simulink model "qa_old_models"  (Simulink 7.3)
settings: Solver=ode45  StartTime=0.0  StopTime=10.0  RelTol=1e-3
values from neighbouring files (symbols this model uses):
  fixpt_adder_out_bitwidth = w    (= 24)    [one_bit_control.m]
  fixpt_adder_out_position = d    (= 16)    [one_bit_control.m]
settings Model: Creator=kunal  LastModifiedBy=kunal

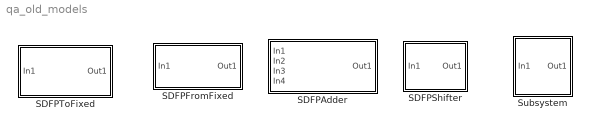
== system qa_old_models ==
  SDFPAdder : Subsystem  mask{in_bitwidth=32, in_fp_position=8, out_bitwidth=32, out_fp_position=8}
      mask prompts: in_bitwidth "Input Bitwidth"; in_fp_position "Input Point Position"; out_bitwidth "Output Bitwidth"; out_fp_position "Output Point Position"
      mask Display: disp(['+\nSDFP'])
  SDFPFromFixed : Subsystem  mask{bitwidth=32, fp_position=16}
      mask prompts: bitwidth "Input Bitwidth"; fp_position "Input Point Position"
      mask Display: disp('Fixed -> Float');
  SDFPShifter : Subsystem  mask{shift_amount=1}
      mask init:
      | if(shift_amount > 0)
      |     dispval=sprintf('<< %d',shift_amount);
      | else
      |     dispval=sprintf('>> %d',-shift_amount);
      | end
      mask Display: disp(dispval);
  SDFPToFixed : Subsystem  mask{bitwidth=fixpt_adder_out_bitwidth, fp_position=fixpt_adder_out_position}
      mask prompts: bitwidth "Output Bitwidth"; fp_position "Output Point Position"
      mask Display: disp('Float -> Fixed')
  Subsystem : Subsystem  mask{gain=1.52, bitwidth=32, fp_position=16}
      mask prompts: bitwidth "Output Bitwidth"; fp_position "Output Point Position"
      mask Display: plot([0.2 0.9 0.2 0.2],[0 .5 1 0]);disp('GainMux')

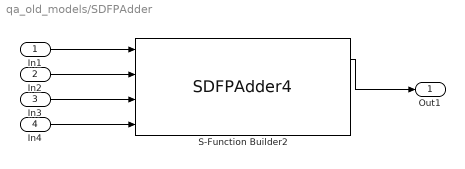
== system qa_old_models/SDFPAdder ==
  In1 : Inport  OutDataType=fixdt(1, 16)  OutScaling=2^0
  In2 : Inport  Port=2  OutDataType=fixdt(1, 16)  OutScaling=2^0
  In3 : Inport  Port=3  OutDataType=fixdt(1, 16)  OutScaling=2^0
  In4 : Inport  Port=4  OutDataType=fixdt(1, 16)  OutScaling=2^0
  S-Function Builder2 : S-Function  InitFcn=try, set_param(gcb,'FunctionName','SDFPAdder4'), end  FunctionName=SDFPAdder4  Parameters=uint32(in_bitwidth),uint32(in_fp_position),uint32(out_bitwidth),uint32(out_fp_position)  SFunctionModules=SDFPAdder4_wrapper  WizardData=DataTag0  EnableBusSupport=off  mask(S-Function Builder){}
      mask help: The S-Function Builder block creates a wrapper C-MEX S-function from your supplied C code with multiple input ports, output ports, and a variable number of scalar, vector, or matrix parameters. The input and output ports can propagate Simulink built-in data types, fixed-point datatypes, complex, frame, 1-D, and 2-D signals. This block also supports discrete and continuous states of type real. You can optionally have the block generate a TLC file to be used with Real-Time Workshop for code generation.
      mask init:
      | val = [[.9  0.75 0.75 1 1 .9 .9 1]',[1 1 0.75 0.75 .9 .9 1 .9]'];try , sys = get_param(gcb,'SfunBuilderFcnName');if isempty(sys), sys = get_param(gcb,'FunctionName'); end,catch, sys = get_param(gcb,'FunctionName'); end
      settings: CopyFcn=set_param(gcbh,'LinkStatus','none')  PreSaveFcn=try, set_param(gcb,'FunctionName','SDFPAdder4'), end  OpenFcn=sfunctionwizard(gcbh)
      mask Display: plot(val(:,1),val(:,2)),disp(sys)port_label('input',1,'in0')port_label('input',2,'in1')port_label('input',3,'in2')port_label('input',4,'in3')port_label('output',1,'adder_out')
  Out1 : Outport  OutDataType=fixdt(1, 16)  OutScaling=2^0
  wires:
  In1/1 -> S-Function Builder2/1
  In2/1 -> S-Function Builder2/2
  In3/1 -> S-Function Builder2/3
  In4/1 -> S-Function Builder2/4
  S-Function Builder2/1 -> Out1/1

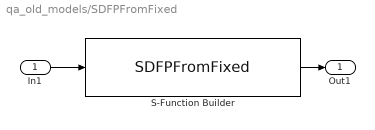
== system qa_old_models/SDFPFromFixed ==
  In1 : Inport  OutDataType=fixdt(1, 16)  OutScaling=2^0
  S-Function Builder : S-Function  InitFcn=try, set_param(gcb,'FunctionName','SDFPFromFixed'), end  FunctionName=SDFPFromFixed  Parameters=uint32(bitwidth),uint32(fp_position)  SFunctionModules=SDFPFromFixed_wrapper fpconv  WizardData=DataTag1  EnableBusSupport=off  mask(S-Function Builder){}
      mask help: The S-Function Builder block creates a wrapper C-MEX S-function from your supplied C code with multiple input ports, output ports, and a variable number of scalar, vector, or matrix parameters. The input and output ports can propagate Simulink built-in data types, fixed-point datatypes, complex, frame, 1-D, and 2-D signals. This block also supports discrete and continuous states of type real. You can optionally have the block generate a TLC file to be used with Real-Time Workshop for code generation.
      mask init: same as qa_old_models/SDFPAdder/S-Function Builder2
      settings: CopyFcn=set_param(gcbh,'LinkStatus','none')  PreSaveFcn=try, set_param(gcb,'FunctionName','SDFPFromFixed'), end  OpenFcn=sfunctionwizard(gcbh)
      mask Display: plot(val(:,1),val(:,2)),disp(sys)port_label('input',1,'fixed_in')port_label('output',1,'float_out')
  Out1 : Outport  OutDataType=fixdt(1, 16)  OutScaling=2^0
  wires:
  In1/1 -> S-Function Builder/1
  S-Function Builder/1 -> Out1/1

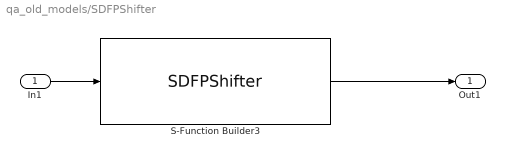
== system qa_old_models/SDFPShifter ==
  In1 : Inport  OutDataType=fixdt(1, 16)  OutScaling=2^0
  S-Function Builder3 : S-Function  InitFcn=try, set_param(gcb,'FunctionName','SDFPShifter'), end  FunctionName=SDFPShifter  Parameters=int32(shift_amount)  SFunctionModules=SDFPShifter_wrapper  WizardData=DataTag2  EnableBusSupport=off  mask(S-Function Builder){}
      mask help: The S-Function Builder block creates a wrapper C-MEX S-function from your supplied C code with multiple input ports, output ports, and a variable number of scalar, vector, or matrix parameters. The input and output ports can propagate Simulink built-in data types, fixed-point datatypes, complex, frame, 1-D, and 2-D signals. This block also supports discrete and continuous states of type real. You can optionally have the block generate a TLC file to be used with Real-Time Workshop for code generation.
      mask init: same as qa_old_models/SDFPAdder/S-Function Builder2
      settings: CopyFcn=set_param(gcbh,'LinkStatus','none')  PreSaveFcn=try, set_param(gcb,'FunctionName','SDFPShifter'), end  OpenFcn=sfunctionwizard(gcbh)
      mask Display: plot(val(:,1),val(:,2)),disp(sys)port_label('input',1,'sg_in')port_label('output',1,'shifter_out')
  Out1 : Outport  OutDataType=fixdt(1, 16)  OutScaling=2^0
  wires:
  In1/1 -> S-Function Builder3/1
  S-Function Builder3/1 -> Out1/1

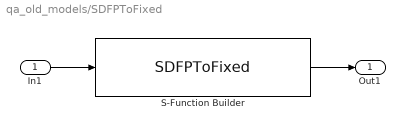
== system qa_old_models/SDFPToFixed ==
  In1 : Inport  OutDataType=fixdt(1, 16)  OutScaling=2^0
  S-Function Builder : S-Function  InitFcn=try, set_param(gcb,'FunctionName','SDFPToFixed'), end  FunctionName=SDFPToFixed  Parameters=uint32(bitwidth),uint32(fp_position)  SFunctionModules=SDFPToFixed_wrapper fpconv  WizardData=DataTag3  EnableBusSupport=off  mask(S-Function Builder){}
      mask help: The S-Function Builder block creates a wrapper C-MEX S-function from your supplied C code with multiple input ports, output ports, and a variable number of scalar, vector, or matrix parameters. The input and output ports can propagate Simulink built-in data types, fixed-point datatypes, complex, frame, 1-D, and 2-D signals. This block also supports discrete and continuous states of type real. You can optionally have the block generate a TLC file to be used with Real-Time Workshop for code generation.
      mask init: same as qa_old_models/SDFPAdder/S-Function Builder2
      settings: CopyFcn=set_param(gcbh,'LinkStatus','none')  PreSaveFcn=try, set_param(gcb,'FunctionName','SDFPToFixed'), end  OpenFcn=sfunctionwizard(gcbh)
      mask Display: plot(val(:,1),val(:,2)),disp(sys)port_label('input',1,'float_in')port_label('output',1,'fixed_out')
  Out1 : Outport  OutDataType=fixdt(1, 16)  OutScaling=2^0
  wires:
  In1/1 -> S-Function Builder/1
  S-Function Builder/1 -> Out1/1

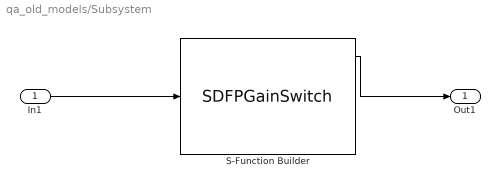
== system qa_old_models/Subsystem ==
  In1 : Inport  OutDataType=fixdt(1, 16)  OutScaling=2^0
  S-Function Builder : S-Function  InitFcn=try, set_param(gcb,'FunctionName','SDFPGainSwitch'), end  FunctionName=SDFPGainSwitch  Parameters=single(gain),uint32(bitwidth),uint32(fp_position)  SFunctionModules=SDFPGainSwitch_wrapper fpconv  WizardData=DataTag4  EnableBusSupport=off  mask(S-Function Builder){}
      mask help: The S-Function Builder block creates a wrapper C-MEX S-function from your supplied C code with multiple input ports, output ports, and a variable number of scalar, vector, or matrix parameters. The input and output ports can propagate Simulink built-in data types, fixed-point datatypes, complex, frame, 1-D, and 2-D signals. This block also supports discrete and continuous states of type real. You can optionally have the block generate a TLC file to be used with Real-Time Workshop for code generation.
      mask init: same as qa_old_models/SDFPAdder/S-Function Builder2
      settings: CopyFcn=set_param(gcbh,'LinkStatus','none')  PreSaveFcn=try, set_param(gcb,'FunctionName','SDFPGainSwitch'), end  OpenFcn=sfunctionwizard(gcbh)
      mask Display: plot(val(:,1),val(:,2)),disp(sys)port_label('input',1,'sd_in')port_label('output',1,'gain_out')
  Out1 : Outport  OutDataType=fixdt(1, 16)  OutScaling=2^0
  wires:
  S-Function Builder/1 -> Out1/1
  In1/1 -> S-Function Builder/1
